simulink model "serial_comms_to_IMU"  (Simulink 7.8)
settings: Solver=FixedStepDiscrete  StartTime=0.0  StopTime=inf  RelTol=1e-3
libraries: xpcseriallib x3, simulink x1, xpclib x1
settings Model: Creator=KTmp  LastModifiedBy=kevinsg  SimulationMode=external  TunableVars=i  TunableVarsStorageClass=Auto  BufferReuse=off
settings DataIOCC: LimitDataPoints=off
settings OptimizationCC: BlockReduction=off  OptimizeBlockIOStorage=off  BufferReuse=off  ExpressionFolding=off  LocalBlockOutputs=off
settings HardwareCC: ProdIntDivRoundTo=Zero  ProdEndianess=LittleEndian  ProdHWDeviceType=Generic->32-bit x86 compatible
settings RTWCC: SystemTargetFile=xpctarget.tlc  TemplateMakefile=xpc_default_tmf  Description=xPC Target  ProcessScript=xpctarget_make_rtw_hook  RTWCompilerOptimization=On
settings xpcTargetCC: TargetFcnLib=ansi_tfl_table_tmw.mat  TargetFunctionLibrary=XPC_BLAS  CodeExecutionProfiling=off  ParMdlRefBuildCompliant=on  ConcurrentExecutionCompliant=on  CombineSignalStateStructs=off  PortableWordSizes=off  RL32LogBufSizeModifier=45000000  xPCTaskExecutionProfile=off  xPCRL32EventNumber=5000  xPCLoadParamSetFile=off  xPCConcurrentTasks=off  xPCEnableSFAnimation=off

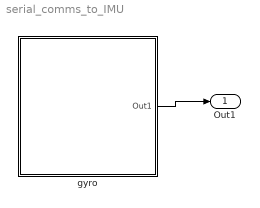
== system serial_comms_to_IMU ==
  gyro : Subsystem
  Out1 : Outport
  wires:
  gyro/1(Out1) -> Out1/1

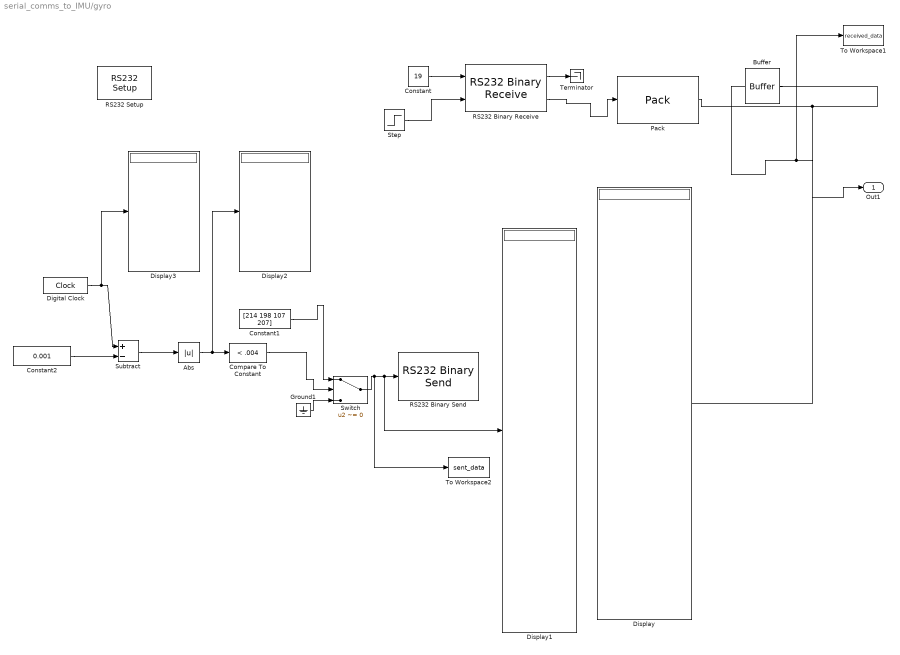
== system serial_comms_to_IMU/gyro ==
  Abs : Abs
  Buffer : Buffer  N=19  TreatMby1Signals=One channel
  Compare To Constant : simulink/Logic and Bit Operations/Compare To Constant  relop=<  const=.004  OutDataTypeStr=boolean  ZeroCross=off
  Constant : Constant  Value=19
  Constant1 : Constant  Value=[214 198 107 207]  OutDataTypeStr=uint8
  Constant2 : Constant  Value=0.001  SampleTime=-1
  Digital Clock : DigitalClock  SampleTime=-1
  Display{,1..3} (4 alike) : Display
  Ground1 : Ground
  Pack : xpclib/UDP/Pack  datatypes={'uint8'}  byteAlign=1
  RS232 Binary Receive : xpcseriallib/Obsolete/Binary Mode/RS232 Binary Receive  port=COM1  width=19  samptime=0.001
  RS232 Binary Send : xpcseriallib/Obsolete/Binary Mode/RS232 Binary Send  port=COM1  width=4  samptime=-1
  "RS232 Setup " : xpcseriallib/Obsolete/RS232 Setup   port=COM1  baud=115200  dbits=8  sbits=1  parity=None  prot=None  sbuf=512  rbuf=512  initstruct=[]  termstruct=[]
  Step : Step  Time=0.004  SampleTime=0.001
  Subtract : Sum  Inputs=+-
  Switch : Switch  Criteria=u2 ~= 0
  Terminator : Terminator
  To Workspace1 : ToWorkspace  VariableName=received_data  SampleTime=-1  SaveFormat=Array
  To Workspace2 : ToWorkspace  VariableName=sent_data  SampleTime=-1  SaveFormat=Array
  Out1 : Outport
  wires:
  Constant/1 -> RS232 Binary Receive/1
  RS232 Binary Receive/2 -> Pack/1
  Pack/1 -> Buffer/1, Display/1
  RS232 Binary Receive/1 -> Terminator/1
  Buffer/1 -> Out1/1, To Workspace1/1
  Step/1 -> RS232 Binary Receive/2
  Abs/1 -> Compare To Constant/1, Display2/1
  Subtract/1 -> Abs/1
  Digital Clock/1 -> Display3/1, Subtract/1
  Constant2/1 -> Subtract/2
  Constant1/1 -> Switch/1
  Switch/1 -> To Workspace2/1, RS232 Binary Send/1, Display1/1
  Ground1/1 -> Switch/3
  Compare To Constant/1 -> Switch/2
